simulink model "practice_answer"  (R2017a)
settings: Solver=FixedStepAuto  StartTime=0.0  StopTime=40000  FixedStep=1  RelTol=1e-3
settings Model: Creator=zhiangz  LastModifiedBy=zhiangz

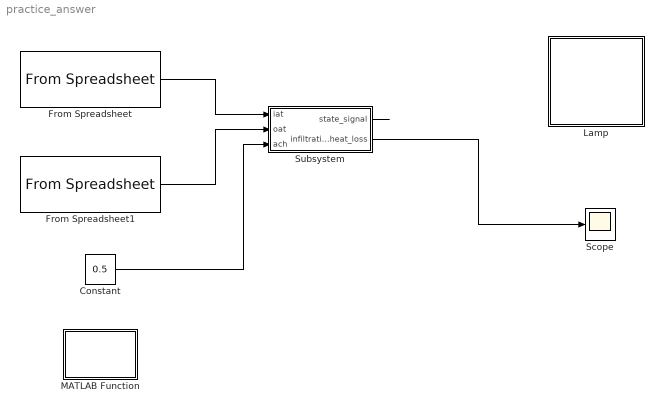
== system practice_answer ==
  Constant : Constant  Value=0.5
  From Spreadsheet : FromSpreadsheet  FileName=indoor_air_temperature.csv  SheetName=indoor_air_temperature  SampleTime=-1
  From Spreadsheet1 : FromSpreadsheet  FileName=outdoor_air_temperature.csv  SheetName=outdoor_air_temperature  SampleTime=-1
  Lamp : Subsystem  DialogController=hmiCreateDDGDialog  IsWebBlock=on  mask(MWDashboardBlock){webBlockId=c2a7fa99-169d-49c1-9f26-a671b7992dc5, webBlockType=lamp, ShowInLibBrowser=on, ShowInitialText=on, HMISrcModelName=practice}
      mask prompts: webBlockType "WebBlock Type"; HMISrcModelName "Source Model"
      mask help: SimulinkHMI:dialogs:LampDialogDesc
      mask Help: helpview([docroot '/mapfiles/simulink.map'], 'hmi_lamp')
      mask Display:
      | if strcmp(get_param(bdroot(gcb),'BlockDiagramType'), 'library')
      |     image([(matlabroot) '/toolbox/simulink/hmi/icons/Lamp.png']);
      | end
  MATLAB Function : MATLAB Function  TreatAsAtomicUnit=on
  Scope : Scope
  Subsystem : Subsystem
  wires:
  From Spreadsheet/1 -> Subsystem/1(iat)
  From Spreadsheet1/1 -> Subsystem/2(oat)
  Subsystem/1(state_signal) -> ?
  Constant/1 -> Subsystem/3(ach)
  Subsystem/2(infiltration_heat_loss) -> Scope/1

== system practice_answer/Lamp ==

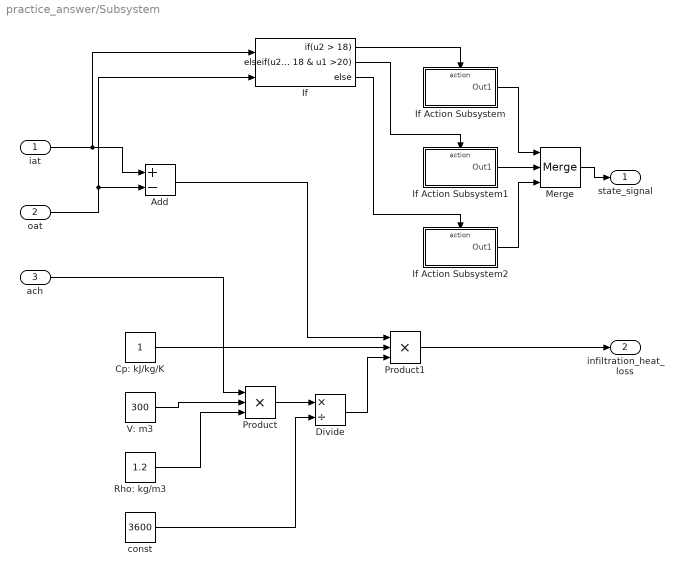
== system practice_answer/Subsystem ==
  iat : Inport
  oat : Inport  Port=2
  ach : Inport  Port=3
  Add : Sum  Inputs=+-
  Cp: kJ/kg/K : Constant
  Divide : Product  Inputs=*/
  If : If  NumInputs=2  IfExpression=u2 > 18  ElseIfExpressions=u2 <= 18 & u1 >20
  If Action Subsystem : Subsystem  TreatAsAtomicUnit=on
  If Action Subsystem1 : Subsystem  TreatAsAtomicUnit=on
  If Action Subsystem2 : Subsystem  TreatAsAtomicUnit=on
  Merge : Merge  Inputs=3
  Product : Product  Inputs=3
  Product1 : Product  Inputs=3
  Rho: kg/m3 : Constant  Value=1.2
  V: m3 : Constant  Value=300
  const : Constant  Value=3600
  state_signal : Outport
  infiltration_heat_loss : Outport  Port=2
  wires:
  Rho: kg/m3/1 -> Product/3
  ach/1 -> Product/1
  V: m3/1 -> Product/2
  Product/1 -> Divide/1
  const/1 -> Divide/2
  oat/1 -> If/2, Add/2
  iat/1 -> If/1, Add/1
  Cp: kJ/kg/K/1 -> Product1/2
  Divide/1 -> Product1/3
  Add/1 -> Product1/1
  Product1/1 -> infiltration_heat_loss/1
  If/1 -> If Action Subsystem/Action
  If/2 -> If Action Subsystem1/Action
  If/3 -> If Action Subsystem2/Action
  If Action Subsystem/1(Out1) -> Merge/1
  If Action Subsystem1/1(Out1) -> Merge/2
  If Action Subsystem2/1(Out1) -> Merge/3
  Merge/1 -> state_signal/1

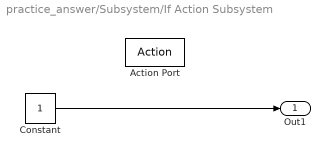
== system practice_answer/Subsystem/If Action Subsystem ==
  Action Port : ActionPort  ActionType=then
  Constant : Constant
  Out1 : Outport
  wires:
  Constant/1 -> Out1/1

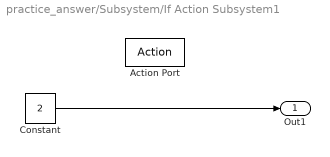
== system practice_answer/Subsystem/If Action Subsystem1 ==
  Action Port : ActionPort  ActionType=elseif
  Constant : Constant  Value=2
  Out1 : Outport
  wires:
  Constant/1 -> Out1/1

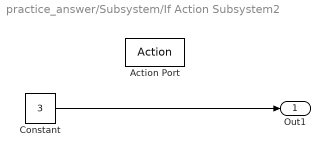
== system practice_answer/Subsystem/If Action Subsystem2 ==
  Action Port : ActionPort  ActionType=else
  Constant : Constant  Value=3
  Out1 : Outport
  wires:
  Constant/1 -> Out1/1

== matlab function practice_answer/MATLAB Function ==
function fcn
pause(0.001);
